simulink model "A2"  (R2023b)
settings: Solver=FixedStepAuto  StartTime=0.0  StopTime=100  FixedStep=1e-3  RelTol=1e-3  EnableMultiTasking=on
undefined symbols (not defined in the file or in its folder): A0, A1, D0, D1, D10, D11, D12, D13, D2, D3, D4, D5, D6, D7, D8, D9, PTA0, PTA1, PTA2, PTB2, PTB23, PTB3, PTB9, PTC16, PTC17, PTC2, PTC3, PTC4, PTD0, PTD1, PTD2, PTD3
libraries: frdmk64flib x20, etargetslib x2, dspstat3 x1
settings Model: ExtModeTrigDuration=5  Creator=Mathew  LastModifiedBy=himan
settings DataIOCC: InspectSignalLogs=on
settings OptimizationCC: EnhancedBackFolding=on  PassReuseOutputArgsAs=Individual arguments  ZeroExternalMemoryAtStartup=off  ZeroInternalMemoryAtStartup=off  MaxStackSize=64  OptimizeBlockOrder=speed  DifferentSizesBufferReuse=on  OptimizationCustomize=off  EfficientTunableParamExpr=on
settings DebuggingCC: ParameterTunabilityLossMsg=error
settings HardwareCC: ProdBitPerPointer=32  ProdBitPerSizeT=32  ProdBitPerPtrDiffT=32  ProdLargestAtomicInteger=Long  ProdLargestAtomicFloat=Double  ProdWordSize=32  ProdHWDeviceType=ARM Compatible->ARM Cortex
settings SFSimCC: MATLABDynamicMemAlloc=off
settings RTWCC: Description=Embedded Coder  SystemTargetFile=ert.tlc  HardwareBoard=NXP FRDM-K64F  TLCOptions="-aInlineSetEventsForThisBaseRateFcn=TLC_FALSE -aSuppressMultiTaskScheduler=TLC_FALSE  -aRateBasedStepFcn=0"  TemplateMakefile=ert_default_tmf  Toolchain=GNU Tools for ARM Embedded Processors
settings CodeAppCC: ForceParamTrailComments=on  IgnoreCustomStorageClasses=off  OperatorAnnotations=on  SimulinkDataObjDesc=on  SFDataObjDesc=on  InsertBlockDesc=on
settings ERTTargetCC: ExtModeTransport=4  ExtModeMexFile=sendToCommService

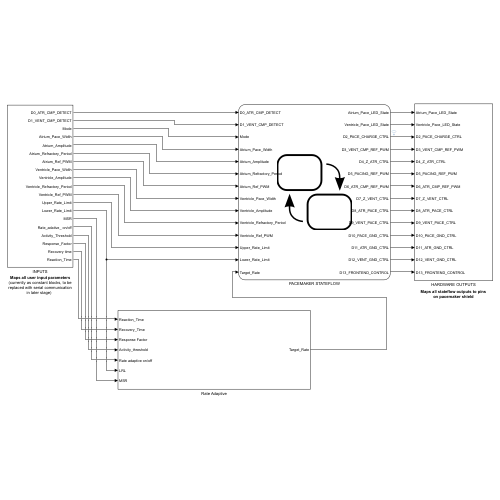
[thumbnail: Simulink's stored preview of the top-level diagram]
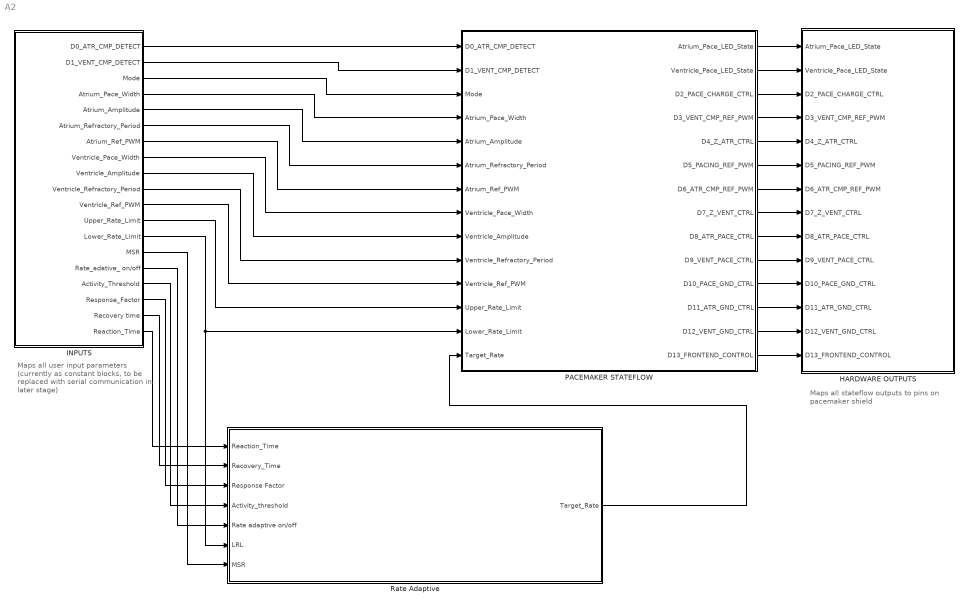
== system A2 ==
  note: Maps all stateflow outputs to pins on pacemaker shield
  note: Maps all user input parameters (currently as constant blocks, to be replaced with serial communication in later stage)
  HARDWARE OUTPUTS : Subsystem
  INPUTS : Subsystem
  PACEMAKER STATEFLOW : Stateflow chart  TreatAsAtomicUnit=on
  Rate Adaptive : Subsystem
  wires:
  INPUTS/6(Atrium_Refractory_Period) -> PACEMAKER STATEFLOW/6(Atrium_Refractory_Period)
  INPUTS/11(Ventricle_Ref_PWM) -> PACEMAKER STATEFLOW/11(Ventricle_Ref_PWM)
  INPUTS/2(D1_VENT_CMP_DETECT) -> PACEMAKER STATEFLOW/2(D1_VENT_CMP_DETECT)
  Rate Adaptive/1(Target_Rate) -> PACEMAKER STATEFLOW/14(Target_Rate)
  INPUTS/12(Upper_Rate_Limit) -> PACEMAKER STATEFLOW/12(Upper_Rate_Limit)
  PACEMAKER STATEFLOW/8(D7_Z_VENT_CTRL) -> HARDWARE OUTPUTS/8(D7_Z_VENT_CTRL)
  PACEMAKER STATEFLOW/1(Atrium_Pace_LED_State) -> HARDWARE OUTPUTS/1(Atrium_Pace_LED_State)
  INPUTS/7(Atrium_Ref_PWM) -> PACEMAKER STATEFLOW/7(Atrium_Ref_PWM)
  PACEMAKER STATEFLOW/3(D2_PACE_CHARGE_CTRL) -> HARDWARE OUTPUTS/3(D2_PACE_CHARGE_CTRL)
  PACEMAKER STATEFLOW/14(D13_FRONTEND_CONTROL) -> HARDWARE OUTPUTS/14(D13_FRONTEND_CONTROL)
  PACEMAKER STATEFLOW/5(D4_Z_ATR_CTRL) -> HARDWARE OUTPUTS/5(D4_Z_ATR_CTRL)
  PACEMAKER STATEFLOW/2(Ventricle_Pace_LED_State) -> HARDWARE OUTPUTS/2(Ventricle_Pace_LED_State)
  PACEMAKER STATEFLOW/9(D8_ATR_PACE_CTRL) -> HARDWARE OUTPUTS/9(D8_ATR_PACE_CTRL)
  INPUTS/8(Ventricle_Pace_Width) -> PACEMAKER STATEFLOW/8(Ventricle_Pace_Width)
  INPUTS/19(Reaction_Time) -> Rate Adaptive/1(Reaction_Time)
  INPUTS/16(Activity_Threshold) -> Rate Adaptive/4(Activity_threshold)
  INPUTS/9(Ventricle_Amplitude) -> PACEMAKER STATEFLOW/9(Ventricle_Amplitude)
  INPUTS/10(Ventricle_Refractory_Period) -> PACEMAKER STATEFLOW/10(Ventricle_Refractory_Period)
  PACEMAKER STATEFLOW/6(D5_PACING_REF_PWM) -> HARDWARE OUTPUTS/6(D5_PACING_REF_PWM)
  INPUTS/5(Atrium_Amplitude) -> PACEMAKER STATEFLOW/5(Atrium_Amplitude)
  INPUTS/4(Atrium_Pace_Width) -> PACEMAKER STATEFLOW/4(Atrium_Pace_Width)
  INPUTS/3(Mode) -> PACEMAKER STATEFLOW/3(Mode)
  INPUTS/15(Rate_adative_ on/off) -> Rate Adaptive/5(Rate adaptive on/off)
  INPUTS/14(MSR) -> Rate Adaptive/7(MSR)
  PACEMAKER STATEFLOW/13(D12_VENT_GND_CTRL) -> HARDWARE OUTPUTS/13(D12_VENT_GND_CTRL)
  PACEMAKER STATEFLOW/11(D10_PACE_GND_CTRL) -> HARDWARE OUTPUTS/11(D10_PACE_GND_CTRL)
  PACEMAKER STATEFLOW/4(D3_VENT_CMP_REF_PWM) -> HARDWARE OUTPUTS/4(D3_VENT_CMP_REF_PWM)
  INPUTS/13(Lower_Rate_Limit) -> PACEMAKER STATEFLOW/13(Lower_Rate_Limit), Rate Adaptive/6(LRL)
  INPUTS/1(D0_ATR_CMP_DETECT) -> PACEMAKER STATEFLOW/1(D0_ATR_CMP_DETECT)
  INPUTS/17(Response_Factor) -> Rate Adaptive/3(Response Factor)
  PACEMAKER STATEFLOW/7(D6_ATR_CMP_REF_PWM) -> HARDWARE OUTPUTS/7(D6_ATR_CMP_REF_PWM)
  PACEMAKER STATEFLOW/12(D11_ATR_GND_CTRL) -> HARDWARE OUTPUTS/12(D11_ATR_GND_CTRL)
  INPUTS/18(Recovery time) -> Rate Adaptive/2(Recovery_Time)
  PACEMAKER STATEFLOW/10(D9_VENT_PACE_CTRL) -> HARDWARE OUTPUTS/10(D9_VENT_PACE_CTRL)

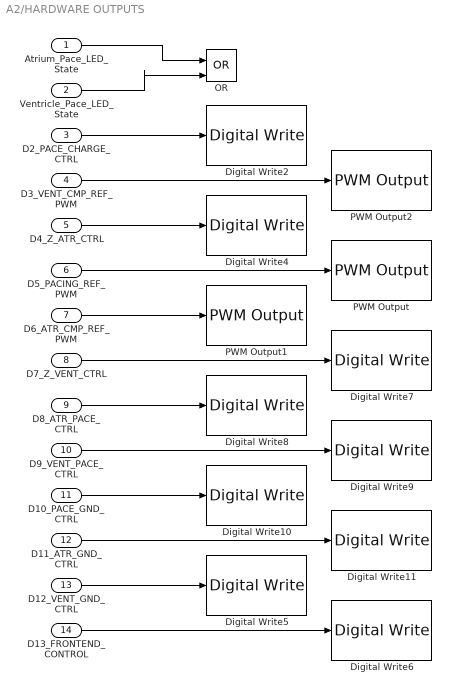
== system A2/HARDWARE OUTPUTS ==
  Atrium_Pace_LED_State : Inport
  Ventricle_Pace_LED_State : Inport  Port=2
  D2_PACE_CHARGE_CTRL : Inport  Port=3
  D3_VENT_CMP_REF_PWM : Inport  Port=4
  D4_Z_ATR_CTRL : Inport  Port=5
  D5_PACING_REF_PWM : Inport  Port=6
  D6_ATR_CMP_REF_PWM : Inport  Port=7
  D7_Z_VENT_CTRL : Inport  Port=8
  D8_ATR_PACE_CTRL : Inport  Port=9
  D9_VENT_PACE_CTRL : Inport  Port=10
  D10_PACE_GND_CTRL : Inport  Port=11
  D11_ATR_GND_CTRL : Inport  Port=12
  D12_VENT_GND_CTRL : Inport  Port=13
  D13_FRONTEND_CONTROL : Inport  Port=14
  Digital Write10 : frdmk64flib/Digital Write  Whichpin=PTD0 (D10)
  Digital Write11 : frdmk64flib/Digital Write  Whichpin=PTD2 (D11)
  Digital Write2 : frdmk64flib/Digital Write  Whichpin=PTB9 (D2)
  Digital Write4 : frdmk64flib/Digital Write  Whichpin=PTB23 (D4)
  Digital Write5 : frdmk64flib/Digital Write  Whichpin=PTD3 (D12)
  Digital Write6 : frdmk64flib/Digital Write  Whichpin=PTD1 (D13)
  Digital Write7 : frdmk64flib/Digital Write  Whichpin=PTC3 (D7)
  Digital Write8 : frdmk64flib/Digital Write  Whichpin=PTA0 (D8)
  Digital Write9 : frdmk64flib/Digital Write  Whichpin=PTC4 (D9)
  OR : Logic  Operator=OR  IconShape=distinctive  AllPortsSameDT=off  OutDataTypeStr=boolean
  PWM Output : frdmk64flib/PWM Output  Whichpin=PTA2 (D5)  InitialFrequency=2000  InitialDutyCycle=0
  PWM Output1 : frdmk64flib/PWM Output  Whichpin=PTC2 (D6)  InitialFrequency=2000  InitialDutyCycle=0
  PWM Output2 : frdmk64flib/PWM Output  Whichpin=PTA1 (D3)  InitialFrequency=2000  InitialDutyCycle=0
  wires:
  D2_PACE_CHARGE_CTRL/1 -> Digital Write2/1
  D3_VENT_CMP_REF_PWM/1 -> PWM Output2/1
  D4_Z_ATR_CTRL/1 -> Digital Write4/1
  D5_PACING_REF_PWM/1 -> PWM Output/1
  D6_ATR_CMP_REF_PWM/1 -> PWM Output1/1
  D7_Z_VENT_CTRL/1 -> Digital Write7/1
  D8_ATR_PACE_CTRL/1 -> Digital Write8/1
  D9_VENT_PACE_CTRL/1 -> Digital Write9/1
  D10_PACE_GND_CTRL/1 -> Digital Write10/1
  D11_ATR_GND_CTRL/1 -> Digital Write11/1
  D12_VENT_GND_CTRL/1 -> Digital Write5/1
  D13_FRONTEND_CONTROL/1 -> Digital Write6/1
  Atrium_Pace_LED_State/1 -> OR/1
  Ventricle_Pace_LED_State/1 -> OR/2

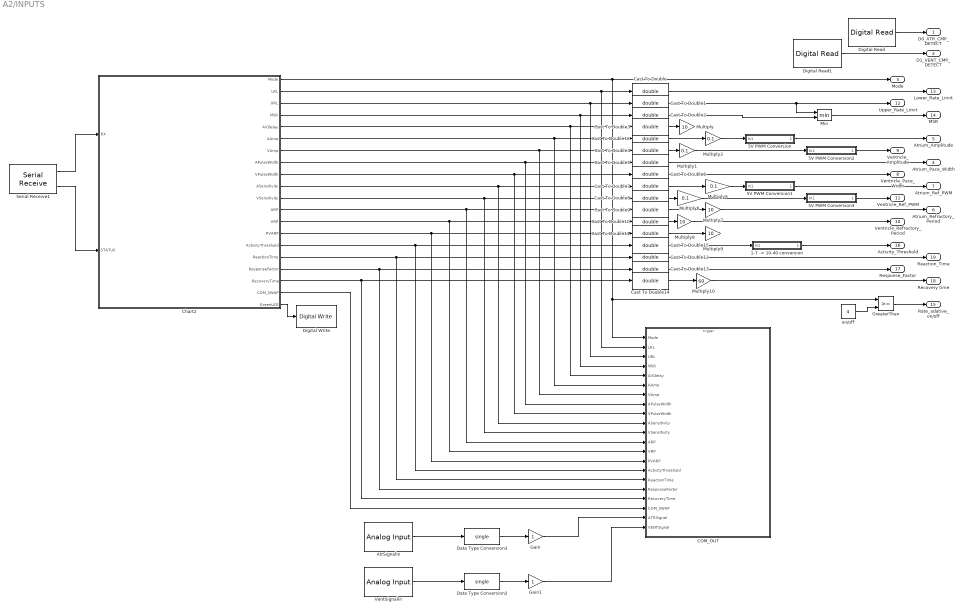
== system A2/INPUTS ==
  "1-7 -> 10-40 conversion" : Subsystem
  5V PWM Conversion : Subsystem
  5V PWM Conversion1 : Subsystem
  5V PWM Conversion2 : Subsystem
  5V PWM Conversion3 : Subsystem
  AtrSignalIn : frdmk64flib/Analog Input  Whichpin=PTB2 (A0)  SampleTime=-1
  "COM_OUT " : Subsystem  TreatAsAtomicUnit=on
  Cast To Double{,1..16} (17 alike) : DataTypeConversion  OutDataTypeStr=double  SaturateOnIntegerOverflow=off  RndMeth=Floor
  Chart2 : Stateflow chart  TreatAsAtomicUnit=on
      settings: PortSchema="{\"entries\":[{\"content\":{\"sides\":[{\"content\":{\"connectorIds\":[\"In1\",\"In2\"]},\"type\":\"ConnectorPlacement.EquallySpacedRectSide\",\"uuid\":\"ffb3d753-dbd9-4cc9-b3f6-be85e99fedf4\"},{\"content\":{\"connectorIds\":[\"Out1\",\"Out2\",\"Out3\",\"Out4\",\"Out5\",\"Out6\",\"Out7\",\"Out8\",\"Out9\",\"Out10\",\"Out11\",\"Out12\",\"Out13\",\"Out14\",\"Out15\",\"Out16\",\"Out17\",\"Out18\",\"Out20\",\"Out19\"],\"side\":\"RIGHT\"},\"type\":\"ConnectorPlacement.EquallySpacedRectSide\",\"uuid\":\"d9281469-7b65-4fbb-b110-42e9dc9d143e\"},{\"content\":{\"side\":\"TOP\"},\"type\":\"ConnectorPlacement.EquallySpacedRectSide\",\"uuid\":\"c04fd83a-1ddb-447c-b8da-2c1ff021f229\"}]},\"type\":\"ConnectorPlacement.EquallySpacedConnector\",\"uuid\":\"b5cd29c2-8e65-48be-b85d-9c735eabd7c7\"}],\"packageUris\":[\"http://schema.mathworks.com/mf0/Connector/R2020b\"],\"version\":\"1.0\"}"
  Data Type Conversion2 : DataTypeConversion  OutDataTypeStr=single  RndMeth=Nearest  SaturateOnIntegerOverflow=off
  Data Type Conversion3 : DataTypeConversion  OutDataTypeStr=single  RndMeth=Nearest  SaturateOnIntegerOverflow=off
  Digital Read : frdmk64flib/Digital Read  Whichpin=PTC16 (D0)  SampleTime=-1
  Digital Read1 : frdmk64flib/Digital Read  Whichpin=PTC17 (D1)  SampleTime=-1
  Digital Write : frdmk64flib/Digital Write  Whichpin=GREEN_LED
  Gain : Gain
  Gain1 : Gain
  GreaterThan : RelationalOperator  OutDataTypeStr=boolean  RndMeth=Simplest  InputSameDT=off
  Min : MinMax  Inputs=2
  Multiply{,7..9} (4 alike) : Gain  Gain=10
  Multiply{1..2,5..6} (4 alike) : Gain  Gain=0.1
  Multiply10 : Gain  Gain=60
  Serial Receive1 : frdmk64flib/Serial Receive  SCIModule=0  Baudrate=uint32(9600)  Parity=None  StopBits=1  HardwareFlowControl=None  ByteOrder=LittleEndian  DataType=uint8  DataLength=20  BlockingMode=off  OutputStatus=on  SampleTime=-1
  VentSignalIn : frdmk64flib/Analog Input  Whichpin=PTB3 (A1)  SampleTime=-1
  on/off : Constant  Value=4
  D0_ATR_CMP_DETECT : Outport
  D1_VENT_CMP_DETECT : Outport  Port=2
  Mode : Outport  Port=3
  Atrium_Pace_Width : Outport  Port=4
  Atrium_Amplitude : Outport  Port=5
  Atrium_Refractory_Period : Outport  Port=6
  Atrium_Ref_PWM : Outport  Port=7
  Ventricle_Pace_Width : Outport  Port=8
  Ventricle_Amplitude : Outport  Port=9
  Ventricle_Refractory_Period : Outport  Port=10
  Ventricle_Ref_PWM : Outport  Port=11
  Upper_Rate_Limit : Outport  Port=12
  Lower_Rate_Limit : Outport  Port=13
  MSR : Outport  Port=14
  Rate_adative_ on/off : Outport  Port=15
  Activity_Threshold : Outport  Port=16
  Response_Factor : Outport  Port=17
  Recovery time : Outport  Port=18
  Reaction_Time : Outport  Port=19
  wires:
  Digital Read/1 -> D0_ATR_CMP_DETECT/1
  Digital Read1/1 -> D1_VENT_CMP_DETECT/1
  Chart2/1(Mode) -> Mode/1, "COM_OUT "/1(Mode), GreaterThan/1
  Chart2/2(LRL) -> "COM_OUT "/2(LRL), Cast To Double/1
  Chart2/3(URL) -> "COM_OUT "/3(URL), Cast To Double1/1
  Chart2/4(MSR) -> "COM_OUT "/4(MSR), Cast To Double2/1
  Serial Receive1/2 -> Chart2/2(STATUS)
  Serial Receive1/1 -> Chart2/1(RX)
  Chart2/7(VAmp) -> "COM_OUT "/7(VAmp), Cast To Double4/1
  Chart2/6(AAmp) -> "COM_OUT "/6(AAmp), Cast To Double16/1
  Chart2/8(APulseWidth) -> "COM_OUT "/8(APulseWidth), Cast To Double5/1
  Chart2/9(VPulseWidth) -> "COM_OUT "/9(VPulseWidth), Cast To Double6/1
  Chart2/10(ASensitivity) -> "COM_OUT "/10(ASensitivity), Cast To Double7/1
  Chart2/11(VSensitivity) -> "COM_OUT "/11(VSensitivity), Cast To Double8/1
  Chart2/12(ARP) -> "COM_OUT "/12(ARP), Cast To Double9/1
  Chart2/13(VRP) -> "COM_OUT "/13(VRP), Cast To Double10/1
  Chart2/14(PVARP) -> "COM_OUT "/14(PVARP), Cast To Double11/1
  Chart2/18(RecoveryTime) -> "COM_OUT "/18(RecoveryTime), Cast To Double14/1
  Chart2/17(ResponseFactor) -> "COM_OUT "/17(ResponseFactor), Cast To Double13/1
  Chart2/16(ReactionTime) -> "COM_OUT "/16(ReactionTime), Cast To Double12/1
  Cast To Double3/1 -> Multiply/1
  Chart2/5(AVDelay) -> "COM_OUT "/5(AVDelay), Cast To Double3/1
  Cast To Double4/1 -> Multiply1/1
  Cast To Double7/1 -> Multiply5/1
  Cast To Double8/1 -> Multiply6/1
  Cast To Double9/1 -> Multiply7/1
  Cast To Double10/1 -> Multiply8/1
  Cast To Double11/1 -> Multiply9/1
  Cast To Double14/1 -> Multiply10/1
  Chart2/15(ActivityThreshold) -> "COM_OUT "/15(ActivityThreshold), Cast To Double15/1
  Cast To Double16/1 -> Multiply2/1
  on/off/1 -> GreaterThan/2
  Chart2/19(GreenLED) -> Digital Write/1
  Data Type Conversion2/1 -> Gain1/1
  Data Type Conversion3/1 -> Gain/1
  AtrSignalIn/1 -> Data Type Conversion3/1
  VentSignalIn/1 -> Data Type Conversion2/1
  Gain/1 -> "COM_OUT "/20(ATRSignal)
  Gain1/1 -> "COM_OUT "/21(VENTSignal)
  Cast To Double/1 -> Lower_Rate_Limit/1
  Cast To Double1/1 -> Min/1, Upper_Rate_Limit/1
  Multiply2/1 -> 5V PWM Conversion/1(In1)
  5V PWM Conversion/1(" ") -> Atrium_Amplitude/1
  5V PWM Conversion2/1(" ") -> Ventricle_Amplitude/1
  Multiply1/1 -> 5V PWM Conversion2/1(In1)
  Cast To Double5/1 -> Atrium_Pace_Width/1
  Cast To Double6/1 -> Ventricle_Pace_Width/1
  Multiply5/1 -> 5V PWM Conversion1/1(In1)
  Multiply6/1 -> 5V PWM Conversion3/1(In1)
  5V PWM Conversion3/1(" ") -> Ventricle_Ref_PWM/1
  5V PWM Conversion1/1(" ") -> Atrium_Ref_PWM/1
  Multiply7/1 -> Atrium_Refractory_Period/1
  Multiply8/1 -> Ventricle_Refractory_Period/1
  Cast To Double12/1 -> Reaction_Time/1
  Cast To Double13/1 -> Response_Factor/1
  Multiply10/1 -> Recovery time/1
  Cast To Double15/1 -> "1-7 -> 10-40 conversion"/1(In1)
  GreaterThan/1 -> Rate_adative_ on/off/1
  Cast To Double2/1 -> Min/2
  Min/1 -> MSR/1
  Chart2/20(COM_SWAP) -> "COM_OUT "/19(COM_SWAP)
  "1-7 -> 10-40 conversion"/1(" ") -> Activity_Threshold/1

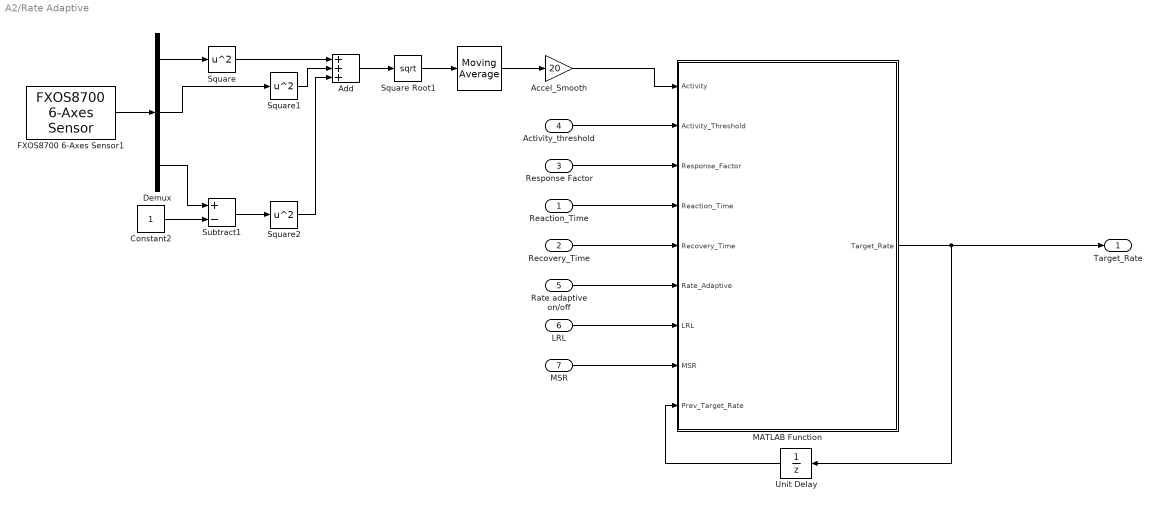
== system A2/Rate Adaptive ==
  Reaction_Time : Inport
  Recovery_Time : Inport  Port=2
  Response Factor : Inport  Port=3
  Activity_threshold : Inport  Port=4
  Rate adaptive on/off : Inport  Port=5
  LRL : Inport  Port=6
  MSR : Inport  Port=7
  " " : dspstat3/Moving Average  Method=Sliding window  ForgettingFactorPort=off  SpecifyWindowLength=on  WindowLength=300  OverlapLength=299  AllowArbitraryInputLength=off  ForgettingFactor=0.9  SimulateUsing=Code generation
  Accel_Smooth : Gain  Gain=20
  Add : Sum  Inputs=+++
  Constant2 : Constant
  Demux : Demux  Outputs=3
  FXOS8700 6-Axes Sensor1 : frdmk64flib/FXOS8700 6-Axes Sensor  Activesensor=Accelerometer only  ODR=800Hz  HybridODR=400Hz  Accelfullrange=-4g to +4g  SampleTime=-1
  MATLAB Function : MATLAB Function  TreatAsAtomicUnit=on
  Square : Math  Operator=square
  Square Root1 : Sqrt
  Square1 : Math  Operator=square
  Square2 : Math  Operator=square
  Subtract1 : Sum  Inputs=+-
  Unit Delay : UnitDelay  SampleTime=-1  HasFrameUpgradeWarning=on
  Target_Rate : Outport
  wires:
  Rate adaptive on/off/1 -> MATLAB Function/6(Rate_Adaptive)
  FXOS8700 6-Axes Sensor1/1 -> Demux/1
  Demux/1 -> Square/1
  Square1/1 -> Add/2
  Square/1 -> Add/1
  Demux/2 -> Square1/1
  Demux/3 -> Subtract1/1
  Constant2/1 -> Subtract1/2
  Subtract1/1 -> Square2/1
  Square2/1 -> Add/3
  Add/1 -> Square Root1/1
  Square Root1/1 -> " "/1
  " "/1 -> Accel_Smooth/1
  Accel_Smooth/1 -> MATLAB Function/1(Activity)
  Activity_threshold/1 -> MATLAB Function/2(Activity_Threshold)
  Recovery_Time/1 -> MATLAB Function/5(Recovery_Time)
  Response Factor/1 -> MATLAB Function/3(Response_Factor)
  LRL/1 -> MATLAB Function/7(LRL)
  Reaction_Time/1 -> MATLAB Function/4(Reaction_Time)
  MSR/1 -> MATLAB Function/8(MSR)
  Unit Delay/1 -> MATLAB Function/9(Prev_Target_Rate)
  MATLAB Function/1(Target_Rate) -> Target_Rate/1, Unit Delay/1

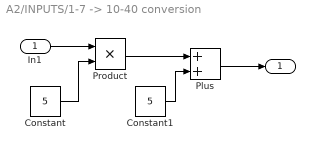
== system A2/INPUTS/1-7 -> 10-40 conversion ==
  In1 : Inport
  Constant : Constant  Value=5
  Constant1 : Constant  Value=5
  Plus : Sum
  Product : Product
  " " : Outport
  wires:
  In1/1 -> Product/1
  Constant/1 -> Product/2
  Product/1 -> Plus/1
  Constant1/1 -> Plus/2
  Plus/1 -> " "/1

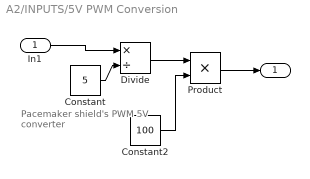
== system A2/INPUTS/5V PWM Conversion ==
  note: Pacemaker shield's PWM 5V converter
  In1 : Inport
  Constant : Constant  Value=5
  Constant2 : Constant  Value=100
  Divide : Product  Inputs=*/
  Product : Product
  " " : Outport
  wires:
  Divide/1 -> Product/1
  Constant2/1 -> Product/2
  Constant/1 -> Divide/2
  In1/1 -> Divide/1
  Product/1 -> " "/1

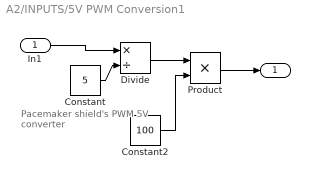
== system A2/INPUTS/5V PWM Conversion1 ==
  note: Pacemaker shield's PWM 5V converter
  In1 : Inport
  Constant : Constant  Value=5
  Constant2 : Constant  Value=100
  Divide : Product  Inputs=*/
  Product : Product
  " " : Outport
  wires:
  Divide/1 -> Product/1
  Constant2/1 -> Product/2
  Constant/1 -> Divide/2
  In1/1 -> Divide/1
  Product/1 -> " "/1

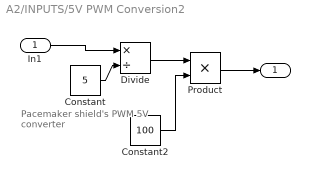
== system A2/INPUTS/5V PWM Conversion2 ==
  note: Pacemaker shield's PWM 5V converter
  In1 : Inport
  Constant : Constant  Value=5
  Constant2 : Constant  Value=100
  Divide : Product  Inputs=*/
  Product : Product
  " " : Outport
  wires:
  Divide/1 -> Product/1
  Constant2/1 -> Product/2
  Constant/1 -> Divide/2
  In1/1 -> Divide/1
  Product/1 -> " "/1

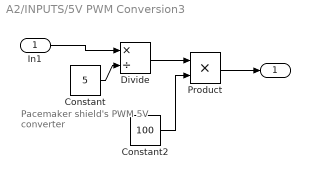
== system A2/INPUTS/5V PWM Conversion3 ==
  note: Pacemaker shield's PWM 5V converter
  In1 : Inport
  Constant : Constant  Value=5
  Constant2 : Constant  Value=100
  Divide : Product  Inputs=*/
  Product : Product
  " " : Outport
  wires:
  Divide/1 -> Product/1
  Constant2/1 -> Product/2
  Constant/1 -> Divide/2
  In1/1 -> Divide/1
  Product/1 -> " "/1

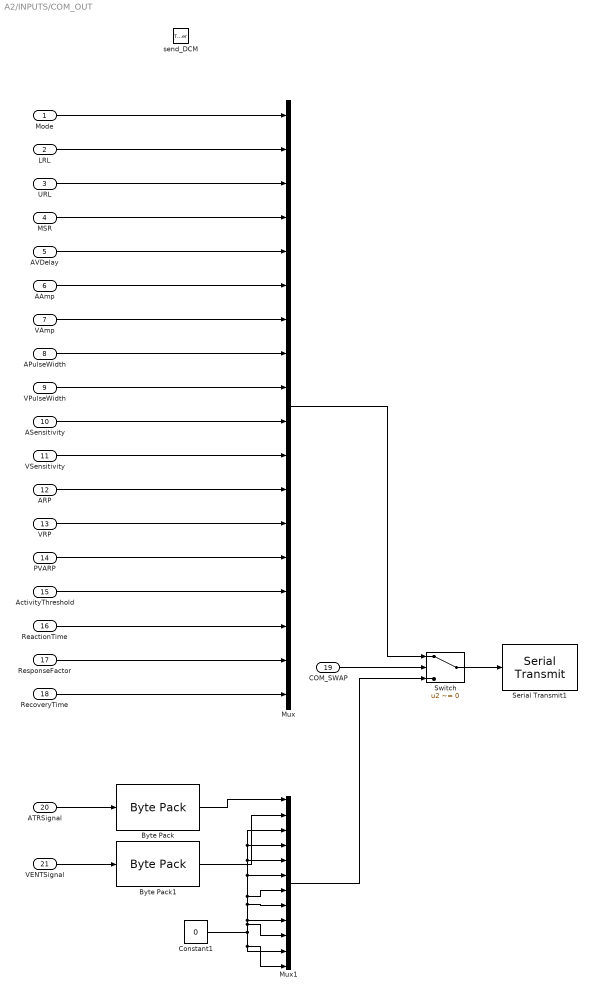
== system A2/INPUTS/COM_OUT  ==
  Mode : Inport
  LRL : Inport  Port=2
  URL : Inport  Port=3
  MSR : Inport  Port=4
  AVDelay : Inport  Port=5
  AAmp : Inport  Port=6
  VAmp : Inport  Port=7
  APulseWidth : Inport  Port=8
  VPulseWidth : Inport  Port=9
  ASensitivity : Inport  Port=10
  VSensitivity : Inport  Port=11
  ARP : Inport  Port=12
  VRP : Inport  Port=13
  PVARP : Inport  Port=14
  ActivityThreshold : Inport  Port=15
  ReactionTime : Inport  Port=16
  ResponseFactor : Inport  Port=17
  RecoveryTime : Inport  Port=18
  COM_SWAP : Inport  Port=19
  ATRSignal : Inport  Port=20
  VENTSignal : Inport  Port=21
  send_DCM : TriggerPort  TriggerType=function-call  IsSimulinkFunction=on  FunctionName=send_DCM  VariantControl=(inherit)
  Byte Pack : etargetslib/Byte Pack  datatypes={'single'}  byteAlign=1
  Byte Pack1 : etargetslib/Byte Pack  datatypes={'single'}  byteAlign=1
  Constant1 : Constant  Value=0  OutDataTypeStr=uint8
  Mux : Mux  Inputs=18
  Mux1 : Mux  Inputs=12
  Serial Transmit1 : frdmk64flib/Serial Transmit  SCIModule=0  Baudrate=uint32(9600)  Parity=None  StopBits=1  HardwareFlowControl=None  ByteOrder=LittleEndian  BlockingMode=on  OutputStatus=off
  Switch : Switch  Criteria=u2 ~= 0  SaturateOnIntegerOverflow=off  InputSameDT=off
  wires:
  PVARP/1 -> Mux/14
  VRP/1 -> Mux/13
  ARP/1 -> Mux/12
  VSensitivity/1 -> Mux/11
  ASensitivity/1 -> Mux/10
  VPulseWidth/1 -> Mux/9
  APulseWidth/1 -> Mux/8
  VAmp/1 -> Mux/7
  AAmp/1 -> Mux/6
  AVDelay/1 -> Mux/5
  MSR/1 -> Mux/4
  URL/1 -> Mux/3
  LRL/1 -> Mux/2
  Mode/1 -> Mux/1
  ActivityThreshold/1 -> Mux/15
  ReactionTime/1 -> Mux/16
  ResponseFactor/1 -> Mux/17
  RecoveryTime/1 -> Mux/18
  COM_SWAP/1 -> Switch/2
  ATRSignal/1 -> Byte Pack/1
  VENTSignal/1 -> Byte Pack1/1
  Mux1/1 -> Switch/3
  Switch/1 -> Serial Transmit1/1
  Mux/1 -> Switch/1
  Byte Pack/1 -> Mux1/1
  Byte Pack1/1 -> Mux1/2
  Constant1/1 -> Mux1/10, Mux1/8, Mux1/7, Mux1/6, Mux1/5, Mux1/4, Mux1/3, Mux1/9, Mux1/12, Mux1/11

== matlab function A2/Rate Adaptive/MATLAB Function ==
  data: Activity input; Activity_Threshold input; Response_Factor input; Reaction_Time input; Recovery_Time input; Rate_Adaptive input; LRL input; MSR input; Prev_Target_Rate input; Target_Rate output
function Target_Rate   = Rate_Response(Activity,Activity_Threshold,Response_Factor,Reaction_Time,Recovery_Time,Rate_Adaptive,LRL,MSR,Prev_Target_Rate)

Activity_diff = Activity-Activity_Threshold;
if(Activity_diff < -10)
    Activity_diff = -10;
end
Activity_Factor = 10*Response_Factor*(Activity_diff); %negative if below threshold

derivative_Activity=diff(Activity);

if(Rate_Adaptive==0)
    BPM_Accel=0;
elseif(derivative_Activity>=0)              %if increasing
    BPM_Accel=Activity_Factor/Reaction_Time;
else                                        %if decreasing
    BPM_Accel=Activity_Factor/Recovery_Time;
end

Target_Rate=BPM_Accel*(1e-3)+Prev_Target_Rate;

if(Target_Rate<LRL)
    Target_Rate=LRL;
elseif(Target_Rate>MSR)
    Target_Rate=MSR;
elseif(Rate_Adaptive==0)
    Target_Rate=LRL;
end

== stateflow chart A2/PACEMAKER STATEFLOW ==
  state AOO
    state Pace
      entry:
      D5_PACING_REF_PWM = 0
      D2_PACE_CHARGE_CTRL=0;
      D10_PACE_GND_CTRL=1;
      D8_ATR_PACE_CTRL=1;
      D11_ATR_GND_CTRL=0;
      D4_Z_ATR_CTRL=0;
      D7_Z_VENT_CTRL=0;
      D12_VENT_GND_CTRL=0;
      D9_VENT_PACE_CTRL=0;
      Atrium_Pace_LED_State=1;
    state Refractory
      entry:
      D10_PACE_GND_CTRL=1;
      D9_VENT_PACE_CTRL=0;
      D4_Z_ATR_CTRL=0;
      D7_Z_VENT_CTRL=0;
      D8_ATR_PACE_CTRL=0;
      D11_ATR_GND_CTRL=1;
      D12_VENT_GND_CTRL=0;
      D2_PACE_CHARGE_CTRL=1;
      D5_PACING_REF_PWM = Atrium_Amplitude
      Atrium_Pace_LED_State=0;
      Standby_Period=(1/(Target_Rate))*30000
    (default) -> AOO.Refractory
    AOO.Pace -> AOO.Refractory : [after(Atrium_Pace_Width,msec)]
    AOO.Refractory -> AOO.Pace : [after(Standby_Period,msec)]
  state AAI
    state Pace
      entry:
      D5_PACING_REF_PWM = 0
      D2_PACE_CHARGE_CTRL=0;
      D10_PACE_GND_CTRL=1;
      D8_ATR_PACE_CTRL=1;
      D11_ATR_GND_CTRL=0;
      D4_Z_ATR_CTRL=0;
      D7_Z_VENT_CTRL=0;
      D12_VENT_GND_CTRL=0;
      D9_VENT_PACE_CTRL=0;
      Atrium_Pace_LED_State=1;
    state Refractory
      entry:
      D5_PACING_REF_PWM = Atrium_Amplitude
      D10_PACE_GND_CTRL=1;
      D9_VENT_PACE_CTRL=0;
      D4_Z_ATR_CTRL=0;
      D7_Z_VENT_CTRL=0;
      D8_ATR_PACE_CTRL=0;
      D11_ATR_GND_CTRL=1;
      D12_VENT_GND_CTRL=0;
      D2_PACE_CHARGE_CTRL=1;
      D6_ATR_CMP_REF_PWM = Atrium_Ref_PWM;
      Atrium_Pace_LED_State=0;
      Standby_Period=30000/(Target_Rate)
    state waiting
    state Sense
    AAI.Pace -> AAI.Refractory : [after(Atrium_Pace_Width,msec)]
    (default) -> AAI.Refractory
    waiting -> Sense [order 1] : [[after(Atrium_Refractory_Period,msec)]]
    AAI.Refractory -> waiting
    waiting -> waiting [order 2] : [D0_ATR_CMP_DETECT == 1]
    Sense -> waiting [order 2] : [D0_ATR_CMP_DETECT == 1]
    Sense -> AAI.Pace [order 1] : after(Standby_Period-Atrium_Pace_Width-Atrium_Refractory_Period,msec)
  state VOO
    state Pace
      entry:
      D5_PACING_REF_PWM = 0
      D2_PACE_CHARGE_CTRL=0;
      D10_PACE_GND_CTRL=1;
      D8_ATR_PACE_CTRL=0;
      D11_ATR_GND_CTRL=0;
      D4_Z_ATR_CTRL=0;
      D7_Z_VENT_CTRL=0;
      D12_VENT_GND_CTRL=0;
      D9_VENT_PACE_CTRL=1;
      Ventricle_Pace_LED_State=1;
    state Refractory
      entry:
      D10_PACE_GND_CTRL=1;
      D9_VENT_PACE_CTRL=0;
      D4_Z_ATR_CTRL=0;
      D7_Z_VENT_CTRL=0;
      D8_ATR_PACE_CTRL=0;
      D11_ATR_GND_CTRL=0;
      D12_VENT_GND_CTRL=1;
      D2_PACE_CHARGE_CTRL=1;
      D5_PACING_REF_PWM = Ventricle_Amplitude
      Ventricle_Pace_LED_State=0;
      Standby_Period=(1/(Target_Rate))*30000
    (default) -> VOO.Refractory
    VOO.Pace -> VOO.Refractory : [after(Ventricle_Pace_Width,msec)]
    VOO.Refractory -> VOO.Pace : [after(Standby_Period,msec)]
  state VVI
    state Pace1
      entry:
      D5_PACING_REF_PWM = 0
      D2_PACE_CHARGE_CTRL=0;
      D10_PACE_GND_CTRL=1;
      D8_ATR_PACE_CTRL=0;
      D11_ATR_GND_CTRL=0;
      D4_Z_ATR_CTRL=0;
      D7_Z_VENT_CTRL=0;
      D12_VENT_GND_CTRL=0;
      D9_VENT_PACE_CTRL=1;
      Atrium_Pace_LED_State=1;
    state Refractory1
      entry:
      D5_PACING_REF_PWM = Ventricle_Amplitude
      D10_PACE_GND_CTRL=1;
      D9_VENT_PACE_CTRL=0;
      D4_Z_ATR_CTRL=0;
      D7_Z_VENT_CTRL=0;
      D8_ATR_PACE_CTRL=0;
      D11_ATR_GND_CTRL=0;
      D12_VENT_GND_CTRL=1;
      D2_PACE_CHARGE_CTRL=1;
      D3_VENT_CMP_REF_PWM = Ventricle_Ref_PWM;
      Ventricle_Pace_LED_State=0;
      Standby_Period=30000/(Target_Rate)
    state waiting1
    state Sense1
    Pace1 -> Refractory1 : [after(Ventricle_Pace_Width,msec)]
    (default) -> Refractory1
    waiting1 -> Sense1 [order 1] : [[after(Ventricle_Refractory_Period,msec)]]
    Refractory1 -> waiting1
    waiting1 -> waiting1 [order 2] : [D1_VENT_CMP_DETECT == 1]
    Sense1 -> waiting1 [order 2] : [D1_VENT_CMP_DETECT == 1]
    Sense1 -> Pace1 [order 1] : after(Standby_Period-Ventricle_Pace_Width-Ventricle_Refractory_Period,msec)
  (default) -> AOO
  AOO -> AAI [order 1] : [Mode==2 || Mode == 6]
  AAI -> AOO [order 2] : [Mode==0 || Mode ==4]
  AOO -> VVI [order 3] : [Mode==3 || Mode == 7]
  VOO -> AAI [order 3] : [Mode==2 || Mode == 6]
  VOO -> AOO [order 1] : [Mode==0 || Mode == 4]
  AOO -> VOO [order 2] : [Mode==1 || Mode == 5]
  VVI -> AOO [order 3] : [Mode==0 || Mode == 4]
  AAI -> VOO [order 3] : [Mode==1 || Mode == 5]
  VVI -> AAI [order 2] : [Mode==2 || Mode == 6]
  AAI -> VVI [order 1] : [Mode==3 || Mode ==7]
  VOO -> VVI [order 2] : [Mode==3 || Mode == 7]
  VVI -> VOO [order 1] : [Mode==1 || Mode == 5]
  data: D0_ATR_CMP_DETECT input; D1_VENT_CMP_DETECT input; Mode input; Atrium_Pace_Width input; Atrium_Amplitude input; Atrium_Refractory_Period input; Atrium_Ref_PWM input; Ventricle_Pace_Width input; Ventricle_Amplitude input; Ventricle_Refractory_Period input; Ventricle_Ref_PWM input; Atrium_Pace_LED_State output; Ventricle_Pace_LED_State output; D2_PACE_CHARGE_CTRL output; D3_VENT_CMP_REF_PWM output; D4_Z_ATR_CTRL output; D5_PACING_REF_PWM output; D6_ATR_CMP_REF_PWM output; D7_Z_VENT_CTRL output; D8_ATR_PACE_CTRL output; D9_VENT_PACE_CTRL output; D10_PACE_GND_CTRL output; D11_ATR_GND_CTRL output; D12_VENT_GND_CTRL output; Upper_Rate_Limit input; Lower_Rate_Limit input; Standby_Period local; D13_FRONTEND_CONTROL output boolean =true; Target_Rate input

== stateflow chart A2/INPUTS/Chart2 ==
  state Send_EGRAM
    entry:
    COM_SWAP=0;
    send_DCM();
    GreenLED=true;
    exit:
    COM_SWAP=1;
    GreenLED=false;
  state Default
    entry:
    Mode=0;   %int unit8
    LRL=60;   %BPM uint8
    URL=120;   %BPM uint8
    MSR=120;   %BPM uint8
    AVDelay=150;   %ms uint8
    AAmp=50   %V single
    VAmp=50;   %V single
    APulseWidth=1;   %ms single
    VPulseWidth=1;   %ms single
    ASensitivity=40;   %mV single
    VSensitivity=40;   %mV single
    ARP=25;   %ms uint16
    VRP=32;   %ms uint16
    PVARP=32;   %ms uint16
    ActivityThreshold=4;   %int uint8
    ReactionTime=30;   %s uint8
    ResponseFactor=8   %int uint8
    RecoveryTime=5;   %min uint8
    GreenLED=false;
    COM_SWAP=1;
  state entry_1
    exit:
    SYNC=RX(1);
    FUNC=RX(2);
    MODEIN=RX(3);
    LRLIN=RX(4);
    URLIN=RX(5);
    MSRIN=RX(6);
    AVDelayIN = RX(7);
    AAmpIN = RX(8);
    VAmpIN = RX(9);
    APulseWidthIN = RX(10);
    VPulseWidthIN = RX(11);
    ASensitivityIN = RX(12);
    VSensitivityIN = RX(13);
    ARPIN = RX(14);
    VRPIN = RX(15);
    PVARPIN = RX(16);
    ActivityThresholdIN = RX(17);
    ReactionTimeIN = RX(18);
    ResponseFactorIN = RX(19);
    RecoveryTimeIN = RX(20);
  state name
  state hehe
    entry:
  state entry_
    Mode=MODEIN;
    LRL=LRLIN;
    URL=URLIN;
    MSR=MSRIN;
    AVDelay = AVDelayIN;
    AAmp= AAmpIN;
    VAmp = VAmpIN;
    APulseWidth = APulseWidthIN;
    VPulseWidth = VPulseWidthIN;
    ASensitivity = ASensitivityIN;
    VSensitivity = VSensitivityIN;
    ARP = ARPIN;
    VRP = VRPIN;
    PVARP = PVARPIN;
    ActivityThreshold = ActivityThresholdIN;
    ReactionTime = ReactionTimeIN;
    ResponseFactor = ResponseFactorIN;
    RecoveryTime = RecoveryTimeIN;
  state WaitBuffer
  state ReturnData
    entry:
    send_DCM();
  Send_EGRAM -> entry_1
  (default) -> Default
  hehe -> Send_EGRAM [order 3] : [FUNC==56]
  Default -> entry_1
  entry_1 -> name : [STATUS==0]
  hehe -> entry_ [order 1] : [FUNC==85]
  name -> hehe : [SYNC==22]
  hehe -> WaitBuffer [order 2] : [FUNC==34]
  WaitBuffer -> ReturnData : [after(20,msec)]
  ReturnData -> entry_1
  entry_ -> entry_1
  data: RX input; Mode output; FUNC local; SYNC local; STATUS input; LRL output; URL output; MSR output; AVDelay output; AAmp output; VAmp output; APulseWidth output; VPulseWidth output; ASensitivity output; VSensitivity output; ARP output; VRP output; PVARP output; LRLIN local; ActivityThreshold output; ReactionTime output; ResponseFactor output; RecoveryTime output; MSRIN local; URLIN local; AAmpIN local; AVDelayIN local; ARPIN local; APulseWidthIN local; ASensitivityIN local; ActivityThresholdIN local; MODEIN local; PVARPIN local; ReactionTimeIN local; RecoveryTimeIN local; ResponseFactorIN local; VAmpIN local; VPulseWidthIN local; VRPIN local; VSensitivityIN local; GreenLED output; COM_SWAP output
